simulink model "heartrate_treadmil"  (Simulink 7.9)
settings: Solver=ode3  StartTime=0.0  StopTime=Tsim  FixedStep=0.25  RelTol=1e-3
values from neighbouring files (symbols this model uses):
  a1 = 1.844    [heartrate.m]
  a2 = 2.747    [heartrate.m]
  a3 = 5.263    [heartrate.m]
  a4 = 0.099    [heartrate.m]
  a5 = 0.068    [heartrate.m]
libraries: simulink x1
settings Model: Creator=jamil  LastModifiedBy=jamil
settings DataIOCC: LimitDataPoints=off

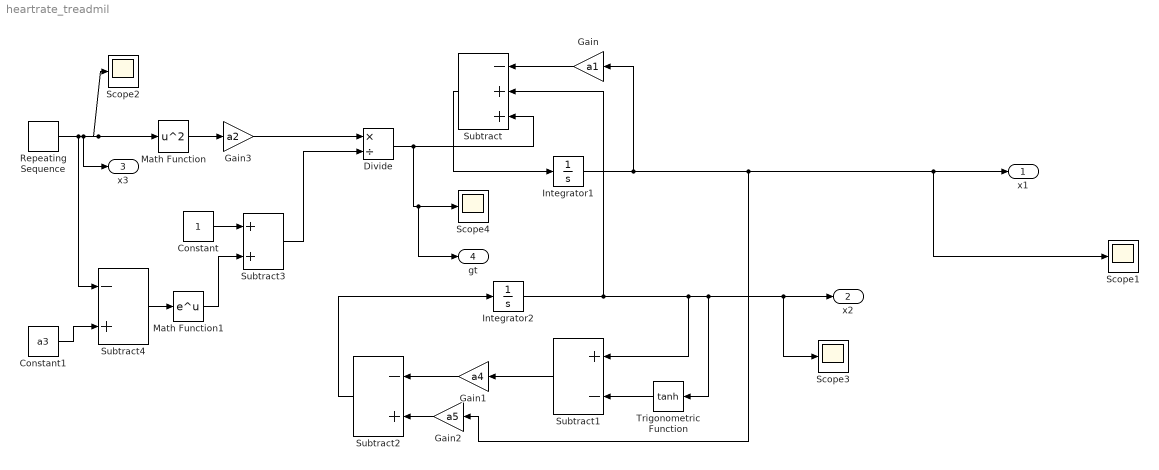
== system heartrate_treadmil ==
  Constant : Constant
  Constant1 : Constant  Value=a3
  Divide : Product  Inputs=*/
  Gain : Gain  Gain=a1
  Gain1 : Gain  Gain=a4
  Gain2 : Gain  Gain=a5
  Gain3 : Gain  Gain=a2
  Integrator1 : Integrator
  Integrator2 : Integrator
  Math Function : Math  Operator=square  SaturateOnIntegerOverflow=on
  Math Function1 : Math  SaturateOnIntegerOverflow=on
  Repeating Sequence : simulink/Sources/Repeating Sequence  rep_seq_t=[0 15 15+1 35]  rep_seq_y=[u u 0 0]
  Scope{1..4} (4 alike) : Scope
      Scope3 settings: SaveName=ScopeData2
      Scope4 settings: SaveName=ScopeData3
  Subtract : Sum  Inputs=-++
  Subtract1 : Sum  Inputs=+-
  Subtract2 : Sum  Inputs=-+
  Subtract3 : Sum
  Subtract4 : Sum  Inputs=-+
  Trigonometric Function : Trigonometry  Operator=tanh
  x1 : Outport
  x2 : Outport  Port=2
  x3 : Outport  Port=3
  gt : Outport  Port=4
  wires:
  Integrator1/1 -> Gain/1, Gain2/1, x1/1, Scope1/1
  Integrator2/1 -> Subtract/2, Subtract1/1, Trigonometric Function/1, x2/1, Scope3/1
  Gain/1 -> Subtract/1
  Subtract1/1 -> Gain1/1
  Trigonometric Function/1 -> Subtract1/2
  Gain1/1 -> Subtract2/1
  Gain2/1 -> Subtract2/2
  Subtract2/1 -> Integrator2/1
  Repeating Sequence/1 -> Subtract4/1, Math Function/1, Scope2/1, x3/1
  Math Function/1 -> Gain3/1
  Gain3/1 -> Divide/1
  Subtract3/1 -> Divide/2
  Constant/1 -> Subtract3/1
  Subtract4/1 -> Math Function1/1
  Math Function1/1 -> Subtract3/2
  Constant1/1 -> Subtract4/2
  Divide/1 -> Subtract/3, Scope4/1, gt/1
  Subtract/1 -> Integrator1/1
